simulink model "SetResetWaitOut"  (Simulink 8.7)
settings: Solver=ode45  StartTime=0.0  StopTime=10.0  RelTol=1e-3
settings Model: Creator=scaife  LastModifiedBy=hamza  ExtModeAutoUpdateStatusClock=off
settings DataIOCC: SaveFormat=Structure  SignalLoggingSaveFormat=ModelDataLogs  SignalLoggingName=sigsOut
settings DebuggingCC: SaveWithParameterizedLinksMsg=none  SignalResolutionControl=TryResolveAllWithWarning  MultiTaskDSMMsg=warning  MultiTaskCondExecSysMsg=none  StrictBusMsg=None
settings HardwareCC: TargetUnknown=on
settings SFSimCC: SimParseCustomCode=off
settings GRTTargetCC: GeneratePreprocessorConditionals=Use local settings  CombineOutputUpdateFcns=off  GRTInterface=on

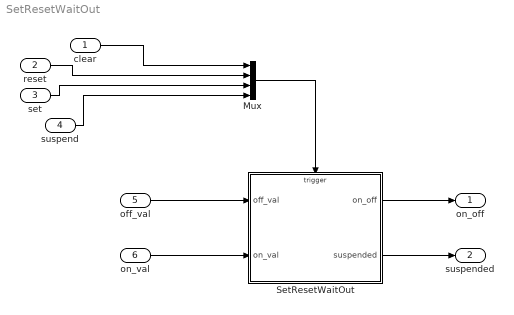
== system SetResetWaitOut ==
  clear : Inport
  reset : Inport  Port=2
  set : Inport  Port=3
  suspend : Inport  Port=4
  off_val : Inport  Port=5
  on_val : Inport  Port=6
  Mux : Mux
  SetResetWaitOut : Stateflow chart  TreatAsAtomicUnit=on
  on_off : Outport
  suspended : Outport  Port=2
  wires:
  off_val/1 -> SetResetWaitOut/1(off_val)
  on_val/1 -> SetResetWaitOut/2(on_val)
  SetResetWaitOut/1(on_off) -> on_off/1
  SetResetWaitOut/2(suspended) -> suspended/1
  Mux/1 -> SetResetWaitOut/Trigger
  clear/1 -> Mux/1
  reset/1 -> Mux/2
  set/1 -> Mux/3
  suspend/1 -> Mux/4

== stateflow chart SetResetWaitOut ==
  state Wait/
    en: suspended=1;
    ex: suspended=0;
  state Off/
    en: on_off=0;
  state On/
    en: on_off=1;
  On -> Wait [order 1] : Suspend
  Off -> On [order 1] : Set
  On -> Off [order 2] : Reset
  Wait -> Off : Clear
  Off -> Wait [order 2] : Suspend
  (default) -> Off
  data: on_off output int32; suspended output uint32; off_val input int32; on_val input int32
  events: Clear input EITHER_EDGE_EVENT; Reset input EITHER_EDGE_EVENT; Set input EITHER_EDGE_EVENT; Suspend input EITHER_EDGE_EVENT
